simulink model "PID-controller(Conti"  (R2018b)
settings: Solver=VariableStepAuto  StartTime=0.0  StopTime=600  RelTol=1e-3
values from neighbouring files (symbols this model uses):
  A = [0 -4.5 0; 0 -0.025 0.000013;0 0 -5.54/60 ]    [Project.m]
  B = [0 0 1/12]'    [Project.m]
  C = [1 0 0]    [Project.m]
  D = -381.1    [Project.m]
  D_bilinear = [D_bilinear;d{1}]    [Project.m]
  D_matched = [D_matched;d{1}]    [Project.m]
  I = -0.0456    [Project.m]
  N_ = 0.07307    [Project.m]
  N_bilinear = [N_bilinear;n{1}]    [Project.m]
  N_matched = [N_matched;n{1}]    [Project.m]
  P = -12.61    [Project.m]
  Ts = [ 0.1 0.9 100]    [Project.m]
libraries: simulink x1
settings Model: Creator=Asus  LastModifiedBy=Asus

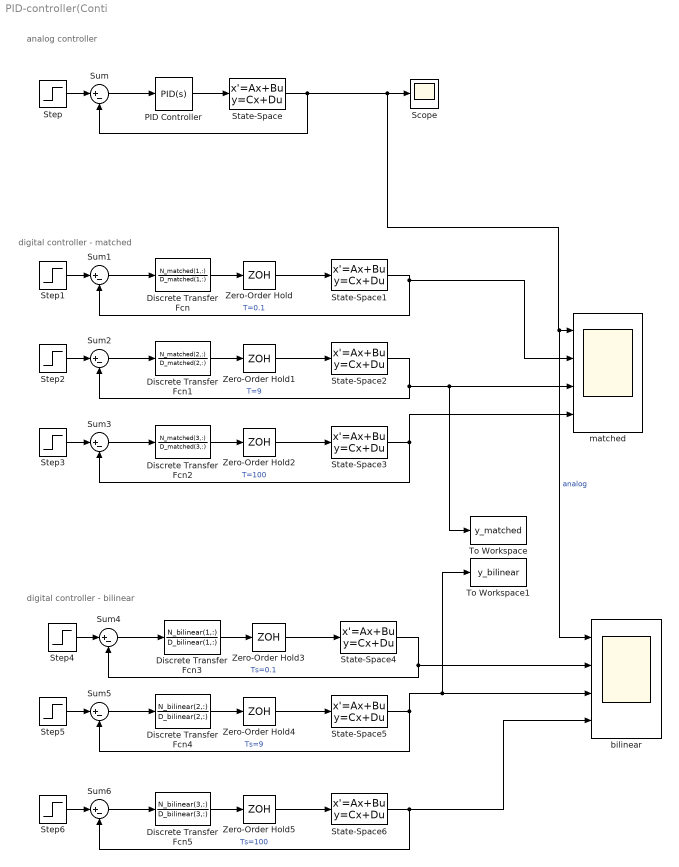
== system PID-controller(Conti ==
  note: analog controller
  note: digital controller - bilinear
  note: digital controller - matched
  Discrete Transfer Fcn : DiscreteTransferFcn  Numerator=N_matched(1,:)  Denominator=D_matched(1,:)
  Discrete Transfer Fcn1 : DiscreteTransferFcn  Numerator=N_matched(2,:)  Denominator=D_matched(2,:)  SampleTime=Ts(2)
  Discrete Transfer Fcn2 : DiscreteTransferFcn  Numerator=N_matched(3,:)  Denominator=D_matched(3,:)  SampleTime=Ts(3)
  Discrete Transfer Fcn3 : DiscreteTransferFcn  Numerator=N_bilinear(1,:)  Denominator=D_bilinear(1,:)  SampleTime=Ts(1)
  Discrete Transfer Fcn4 : DiscreteTransferFcn  Numerator=N_bilinear(2,:)  Denominator=D_bilinear(2,:)  SampleTime=Ts(2)
  Discrete Transfer Fcn5 : DiscreteTransferFcn  Numerator=N_bilinear(3,:)  Denominator=D_bilinear(3,:)  SampleTime=Ts(3)
  PID Controller : simulink/Continuous/PID Controller  Controller=PID  Form=Parallel  TimeDomain=Continuous-time  SampleTime=-1  IntegratorMethod=Forward Euler  FilterMethod=Forward Euler  ControllerParametersSource=internal  P=P  I=I  D=D  UseFilter=on  N=N_  TunerSelectOption=Transfer Function Based (PID Tuner App)  InitialConditionSource=internal  InitialConditionForIntegrator=0  InitialConditionForFilter=0  DifferentiatorICPrevScaledInput=0  ExternalReset=none  TrackingMode=off  Kt=1  LimitOutput=off  UpperSaturationLimit=inf  LowerSaturationLimit=-inf  LinearizeAsGain=on  AntiWindupMode=none  Kb=1  POutMin=[]  POutMax=[]  IOutMin=[]  IOutMax=[]  DOutMin=[]  DOutMax=[]  NOutMin=[]  NOutMax=[]  SumOutMin=[]  SumOutMax=[]  SaturationOutMin=[]  SaturationOutMax=[]  PParamMin=[]  PParamMax=[]  IParamMin=[]  IParamMax=[]  DParamMin=[]  DParamMax=[]  NParamMin=[]  NParamMax=[]  KbParamMin=[]  KbParamMax=[]  KtParamMin=[]  KtParamMax=[]  KbOutMin=[]  KbOutMax=[]  KtOutMin=[]  KtOutMax=[]  IntegratorOutMin=[]  IntegratorOutMax=[]  FilterOutMin=[]  FilterOutMax=[]  SumI1OutMin=[]  SumI1OutMax=[]  SumI2OutMin=[]  SumI2OutMax=[]  SumI3OutMin=[]  SumI3OutMax=[]  SumI4OutMin=[]  SumI4OutMax=[]  SumDOutMin=[]  SumDOutMax=[]  DifferentiatorOutMin=[]  DifferentiatorOutMax=[]  FilterDiffOutCoefMin=[]  FilterDiffOutCoefMax=[]  ReciprocalOutMin=[]  ReciprocalOutMax=[]  SumDenOutMin=[]  SumDenOutMax=[]  SumNumOutMin=[]  SumNumOutMax=[]  DivideOutMin=[]  DivideOutMax=[]  IntegratorContinuousStateAttributes=''  IntegratorStateMustResolveToSignalObject=off  IntegratorRTWStateStorageClass=Auto  FilterContinuousStateAttributes=''  FilterStateMustResolveToSignalObject=off  FilterRTWStateStorageClass=Auto  ParallelPVariant=InternalParameters  IdealPVariant=Disabled  IVariant=InternalParameters  DVariant=InternalParameters  IntegratorVariant=Continuous  SatVariant=Disabled  AWVariant=Passthrough  PCopyVariant=Disabled  TRVariant=Disabled  FdbkBlocksVariant=Forward  IdealPFdbkVariant=Disabled  SatFdbkVariant=Disabled  DerivativeFilterVariant=ContFilter  NVariant=InternalParameters  NCopyVariant=Disabled  FilterICVariant=InternalICsFilter  IntegratorICVariant=InternalICs  ExternalResetVariant=Disabled  TRSumVariant=Passthrough  SumFdbkVariant=Disabled  SumVariant=Sum_PID
  Scope : Scope
  State-Space{,1..6} (7 alike) : StateSpace  A=A  B=B  C=C  D=0  InitialCondition=0
  Step{,1..6} (7 alike) : Step  SampleTime=0
  Sum{,1..6} (7 alike) : Sum  Inputs=|+-
  To Workspace : ToWorkspace  VariableName=y_matched  SaveFormat=Timeseries  SampleTime=-1
  To Workspace1 : ToWorkspace  VariableName=y_bilinear  SaveFormat=Timeseries  SampleTime=-1
  Zero-Order Hold : ZeroOrderHold  SampleTime=Ts(1)
  Zero-Order Hold{1..5} (5 alike) : ZeroOrderHold  SampleTime=-1
  bilinear : Scope  NumInputPorts=4
  "matched " : Scope  NumInputPorts=4
  wires:
  State-Space/1 -> bilinear/1, "matched "/1, Scope/1, Sum/2  "analog"
  Step/1 -> Sum/1
  State-Space1/1 -> "matched "/2, Sum1/2  "T=0.1"
  Sum1/1 -> Discrete Transfer Fcn/1
  Step1/1 -> Sum1/1
  Discrete Transfer Fcn/1 -> Zero-Order Hold/1
  Zero-Order Hold/1 -> State-Space1/1
  Zero-Order Hold1/1 -> State-Space2/1
  Discrete Transfer Fcn1/1 -> Zero-Order Hold1/1
  Step2/1 -> Sum2/1
  Sum2/1 -> Discrete Transfer Fcn1/1
  State-Space2/1 -> To Workspace/1, "matched "/3, Sum2/2  "T=9"
  Zero-Order Hold2/1 -> State-Space3/1
  Discrete Transfer Fcn2/1 -> Zero-Order Hold2/1
  Step3/1 -> Sum3/1
  Sum3/1 -> Discrete Transfer Fcn2/1
  State-Space3/1 -> "matched "/4, Sum3/2  "T=100"
  Zero-Order Hold3/1 -> State-Space4/1
  Discrete Transfer Fcn3/1 -> Zero-Order Hold3/1
  Step4/1 -> Sum4/1
  Sum4/1 -> Discrete Transfer Fcn3/1
  State-Space4/1 -> bilinear/2, Sum4/2  "Ts=0.1"
  State-Space5/1 -> To Workspace1/1, bilinear/3, Sum5/2  "Ts=9"
  Step5/1 -> Sum5/1
  Sum5/1 -> Discrete Transfer Fcn4/1
  Zero-Order Hold4/1 -> State-Space5/1
  Discrete Transfer Fcn4/1 -> Zero-Order Hold4/1
  State-Space6/1 -> bilinear/4, Sum6/2  "Ts=100"
  Step6/1 -> Sum6/1
  Sum6/1 -> Discrete Transfer Fcn5/1
  Zero-Order Hold5/1 -> State-Space6/1
  Discrete Transfer Fcn5/1 -> Zero-Order Hold5/1
  Sum/1 -> PID Controller/1
  PID Controller/1 -> State-Space/1
